simulink model "NA_simple"  (Simulink 7.8)
settings: Solver=FixedStepDiscrete  StartTime=0.0  StopTime=10.0  RelTol=1e-3
settings Model: Creator=medcps  LastModifiedBy=medcps

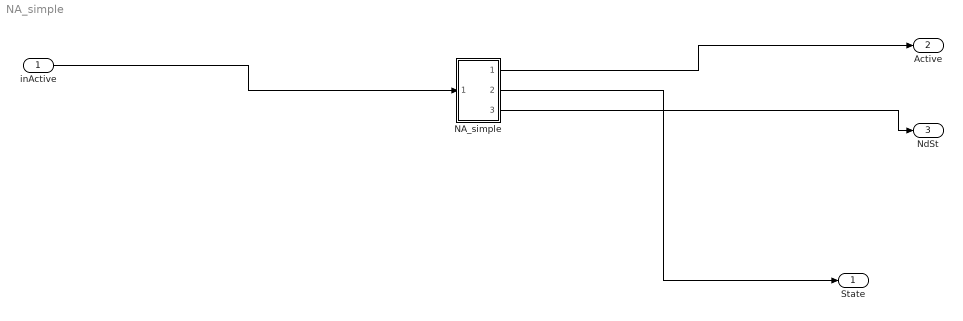
== system NA_simple ==
  inActive : Inport
  NA_simple : Subsystem
  State : Outport
  Active : Outport  Port=2
  NdSt : Outport  Port=3
  wires:
  NA_simple/1(Active) -> Active/1
  inActive/1 -> NA_simple/1(inActive)
  NA_simple/2(State) -> State/1
  NA_simple/3(NdSt) -> NdSt/1

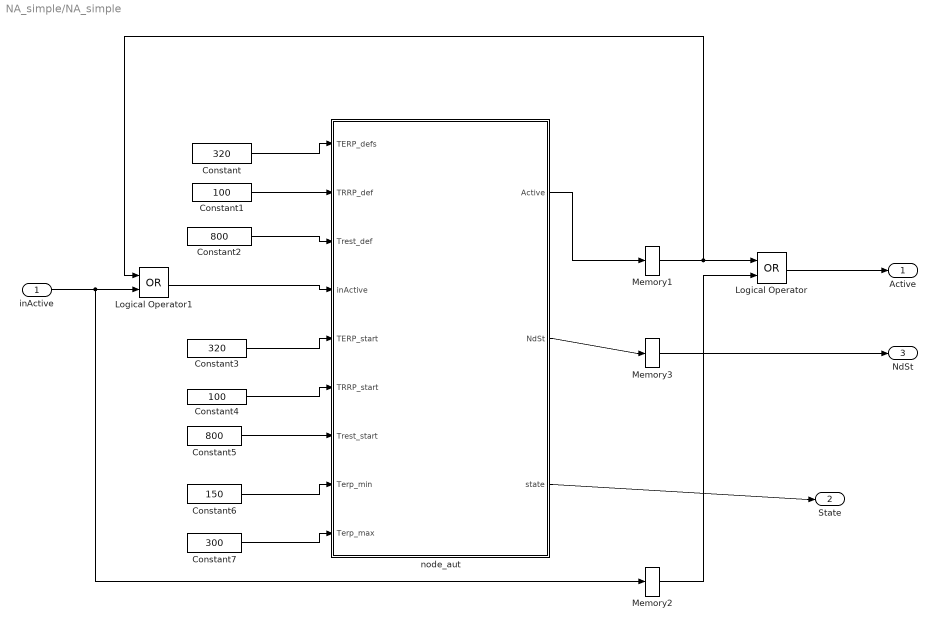
== system NA_simple/NA_simple ==
  inActive : Inport
  Constant : Constant  Value=320  OutDataTypeStr=uint16
  Constant1 : Constant  Value=100  OutDataTypeStr=uint16
  Constant2 : Constant  Value=800  OutDataTypeStr=uint16
  Constant3 : Constant  Value=320  OutDataTypeStr=uint16
  Constant4 : Constant  Value=100  OutDataTypeStr=uint16
  Constant5 : Constant  Value=800  OutDataTypeStr=uint16
  Constant6 : Constant  Value=150  OutDataTypeStr=uint16
  Constant7 : Constant  Value=300  OutDataTypeStr=uint16
  Logical Operator : Logic  Operator=OR  AllPortsSameDT=off  OutDataTypeStr=boolean
  Logical Operator1 : Logic  Operator=OR  AllPortsSameDT=off  OutDataTypeStr=boolean
  Memory1 : Memory  InheritSampleTime=on
  Memory2 : Memory  InheritSampleTime=on
  Memory3 : Memory  InheritSampleTime=on
  node_aut : Stateflow chart  TreatAsAtomicUnit=on
  Active : Outport
  State : Outport  Port=2
  NdSt : Outport  Port=3
  wires:
  Constant/1 -> node_aut/1(TERP_defs)
  Constant1/1 -> node_aut/2(TRRP_def)
  Constant2/1 -> node_aut/3(Trest_def)
  Constant3/1 -> node_aut/5(TERP_start)
  Constant4/1 -> node_aut/6(TRRP_start)
  Constant5/1 -> node_aut/7(Trest_start)
  Constant6/1 -> node_aut/8(Terp_min)
  Constant7/1 -> node_aut/9(Terp_max)
  node_aut/1(Active) -> Memory1/1
  node_aut/2(NdSt) -> Memory3/1
  Memory1/1 -> Logical Operator/1, Logical Operator1/1
  inActive/1 -> Memory2/1, Logical Operator1/2
  Logical Operator1/1 -> node_aut/4(inActive)
  Memory2/1 -> Logical Operator/2
  Logical Operator/1 -> Active/1
  node_aut/3(state) -> State/1
  Memory3/1 -> NdSt/1

== stateflow chart NA_simple/node_aut ==
  settings: executeAtInitialization=1
  state NodeAutomaton
    state Rest
      du: Trest_cur = Trest_cur-1;
      du: state=1;
    state RRP
      du: TRRP_cur = TRRP_cur-1;
      du: state=3;
    state ERP
      ex: Active = 0;
      du: TERP_cur = TERP_cur-1;
      du: NdSt = 0;
      du: Active = 0;
      du: state=2;
    (default) -> Rest : {Active=0;
        | Trest_cur = Trest_start;TERP_def=TERP_defs;
        | TERP_cur = TERP_start;
        | TRRP_cur = TRRP_start;
        | NdSt = 0;}
    Rest -> ERP [order 2] : [inActive]
        | {Trest_cur = Trest_def;
        | TERP_def = Terp_max;
        | TERP_cur = Terp_max;
        | NdSt = 1;}
    ERP -> ERP [order 1] : [inActive]
        | {TERP_cur = Terp_min;
        | TERP_def = Terp_min;
        | NdSt = 2;}
    RRP -> ERP [order 1] : [inActive]
        | {TERP_def = Terp_min;
        | NdSt = 3;
        | TERP_cur = TERP_def;
        | TRRP_cur = TRRP_def;}
    Rest -> ERP [order 1] : [(~inActive)&(Trest_cur==0)]
        | {Trest_cur = Trest_def;
        | Active = 1;NdSt = 0;}
    ERP -> RRP [order 2] : [(~inActive)&(TERP_cur==0)]
        | {TERP_cur = TERP_def;
        | NdSt = 0;}
    RRP -> Rest [order 2] : [(~inActive)&(TRRP_cur==0)]
        | {TRRP_cur = TRRP_def;
        | NdSt = 0;}
  data: TERP_cur local uint16; TRRP_cur local uint16; Trest_cur local uint16; TERP_defs input uint16; TRRP_def input uint16; Trest_def input uint16; Active output boolean; inActive input boolean; TERP_start input uint16; TRRP_start input uint16; Trest_start input uint16; Terp_min input uint16; Terp_max input uint16; NdSt output uint8; TERP_def local uint16; state output uint8
